simulink model "rls"  (R2022b)
settings: Solver=FixedStepAuto  StartTime=0.0  StopTime=910415*Ts  FixedStep=Ts  RelTol=1e-3
PreLoadFcn:
  | gen_workspace
undefined symbols (not defined in the file): Ts
settings Model: Creator=Z153167  LastModifiedBy=Z153167

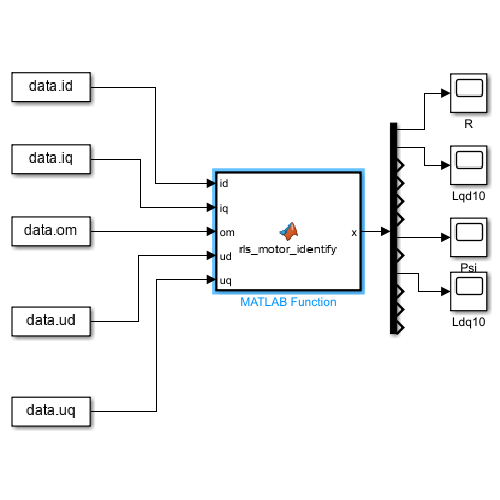
[thumbnail: Simulink's stored preview of the top-level diagram]
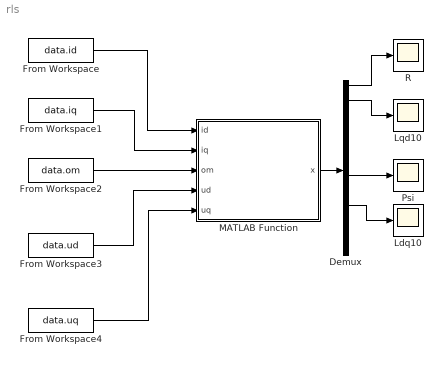
== system rls ==
  Demux : Demux  Outputs=12
  From Workspace : FromWorkspace  VariableName=data.id  SampleTime=Ts  OutputAfterFinalValue=Holding final value
  From Workspace1 : FromWorkspace  VariableName=data.iq  SampleTime=Ts  OutputAfterFinalValue=Holding final value
  From Workspace2 : FromWorkspace  VariableName=data.om  SampleTime=Ts  OutputAfterFinalValue=Holding final value
  From Workspace3 : FromWorkspace  VariableName=data.ud  SampleTime=Ts  OutputAfterFinalValue=Holding final value
  From Workspace4 : FromWorkspace  VariableName=data.uq  SampleTime=Ts  OutputAfterFinalValue=Holding final value
  Ldq10 : Scope
  Lqd10 : Scope
  MATLAB Function : MATLAB Function  TreatAsAtomicUnit=on
  Psi : Scope
  R : Scope
  wires:
  From Workspace2/1 -> MATLAB Function/3(om)
  From Workspace1/1 -> MATLAB Function/2(iq)
  From Workspace3/1 -> MATLAB Function/4(ud)
  From Workspace/1 -> MATLAB Function/1(id)
  From Workspace4/1 -> MATLAB Function/5(uq)
  MATLAB Function/1(x) -> Demux/1
  Demux/7 -> Psi/1
  Demux/1 -> R/1
  Demux/2 -> Lqd10/1
  Demux/9 -> Ldq10/1

== matlab function rls/MATLAB Function ==
  data: id input; x output; iq input; om input; ud input; uq input
function x = rls_motor_identify(id, iq, om, ud, uq)
% RLS_MOTOR_IDENTIFY  Rank-2 Recursive Least Squares parameter identification
%                     for a PMSM motor model, intended for use as a MATLAB
%                     Function block inside Simulink.
%
% USAGE (Simulink MATLAB Function block)
%   - Inputs  : id, iq, om, ud, uq  (all scalar, double)
%   - Output  : x  (12x1 double) — current parameter vector
%
% PARAMETER VECTOR  x  (12 elements, PARAMETER_NAMES order)
%   Index  Name      Axis
%   1      R         d
%   2      Lqd10     d
%   3      Lqd30     d
%   4      Cdq01     d
%   5      Cdq11     d
%   6      R         q   (= x(1) by constraint)
%   7      Psi       q
%   8      Cdq01     q   (= x(4) by constraint)
%   9      Ldq10     q
%   10     Ldq20     q
%   11     Ldq30     q
%   12     Cdq11     q   (= x(5) by constraint)
%
% EQUALITY CONSTRAINTS (enforced via null-space projection)
%   x(1)  == x(6)   (R shared between axes)
%   x(4)  == x(8)   (Cdq01 shared)
%   x(5)  == x(12)  (Cdq11 shared)
%
% ALGORITHM
%   At each time step the function performs one rank-2 RLS update using both
%   the d-axis (Ud) and q-axis (Uq) voltage equations simultaneously.
%   The Woodbury matrix identity is used so that only a cheap 2x2 matrix
%   inversion is required per step.
%   All arithmetic is carried out in the reduced (null-space) coordinate
%   system of dimension r = 9, then mapped back to the full 12-D space.
%
% PERSISTENT STATE
%   Minv  (9x9)  inverse of the reduced normal-equation matrix
%   rhs   (9x1)  reduced right-hand side  Ar' * b  accumulated so far
%   F     (12x9) null-space basis (fixed after first call)
%   x_    (12x1) current full-space parameter estimate

% -------------------------------------------------------------------------
% Persistent variables — survive across Simulink time steps.
% -------------------------------------------------------------------------
persistent Minv rhs F x_

% -------------------------------------------------------------------------
% Constants
% -------------------------------------------------------------------------
N_PARAMS = 12;

% Datasheet / prior-knowledge initial guesses.
start_values = [ ...
    3e-02;  50e-6;  0.;  0.;  0.; ...   % d-axis
    3e-02;  4e-03;  0.; 50e-6;  0.;  0.;  0.];  % q-axis

% Equality constraint pairs
% Each row is [i, j] meaning x(i) must equal x(j).
eq_pairs = [1, 6; 4, 8; 5, 12];  

% Number of synthetic initialisation samples.
N_INIT = 50;

% -------------------------------------------------------------------------
% One-time initialisation (first Simulink call or after a reset).
% -------------------------------------------------------------------------
if isempty(F)
    % --- Build null-space basis F (12 x 9) ---
    n_constraints = size(eq_pairs, 1);   % = 3
    C = zeros(n_constraints, N_PARAMS);
    for k = 1:n_constraints
        C(k, eq_pairs(k,1)) =  1;
        C(k, eq_pairs(k,2)) = -1;
    end
    % null() returns an orthonormal basis for the null space of C.
    F = null(C);   % (12 x 9)

    % --- Bootstrap cache from synthetic data ---
    % Replicate Python's initialise_cache: a linspace grid of 50 (id,iq,om)
    % samples.  The seed is fixed so the initial state is deterministic.
    rng(133);
    id_init  = linspace(-10, 10, N_INIT)' + randn(N_INIT, 1);
    iq_init  = linspace(-10, 10, N_INIT)' + randn(N_INIT, 1);
    om_init  = linspace(-100, 100, N_INIT)' + randn(N_INIT, 1);

    % Build the full (2*N_INIT x 12) design matrix A and target vector b.
    [b_init, A_init] = expand_basis_batch(id_init, iq_init, om_init, ...
                                          zeros(N_INIT,1), zeros(N_INIT,1));
    % Voltages consistent with start_values.
    b_init = A_init * start_values;

    % Project into the reduced space.
    Ar_init = A_init * F;           % (2*N_INIT x 9)
    Minv    = inv(Ar_init' * Ar_init);  % (9 x 9)
    rhs     = Ar_init' * b_init;        % (9 x 1)
    x_      = start_values;             % (12 x 1)
end

% -------------------------------------------------------------------------
% Build the two regressor rows for this time step.
% -------------------------------------------------------------------------
% d-axis row  (5 non-zero entries, columns 1-5):
%   [id,  -om*iq,  -om*iq^3,  -om*id*iq,  -0.5*om*iq*id^2,
%    0,    0,       0,          0,           0,              0, 0]
% q-axis row  (7 non-zero entries, columns 6-12):
%   [0,   0,        0,          0,           0,
%    iq,  om,  0.5*om*iq^2,  om*id,  om*id^2,  om*id^3,  0.5*om*id*iq^2]

a_d = [ id, ...
       -om*iq, ...
       -om*iq^3, ...
       -om*id*iq, ...
       -0.5*om*iq*id^2, ...
        0, 0, 0, 0, 0, 0, 0 ];       % (1 x 12)

a_q = [ 0, 0, 0, 0, 0, ...
        iq, ...
        om, ...
        0.5*om*iq^2, ...
        om*id, ...
        om*id^2, ...
        om*id^3, ...
        0.5*om*id*iq^2 ];             % (1 x 12)

A_new   = [a_d; a_q];        % (2 x 12)
b_new   = [ud; uq];          % (2 x 1)

% -------------------------------------------------------------------------
% Rank-2 RLS update in the reduced space (Woodbury identity).
% -------------------------------------------------------------------------
% Project the two new rows into the reduced space.
Ar_new   = F' * A_new';  % (9 x 2)     

Minv_U   = Minv * Ar_new; % (9 x 2) 

inner    = eye(2) + Ar_new' * Minv_U; % (2 x 2) 

% Explicit 2x2 inversion 
a_i = inner(1,1);  b_i = inner(1,2);
c_i = inner(2,1);  d_i = inner(2,2);
det_val = a_i*d_i - b_i*c_i;

if abs(det_val) < 1e-12
    % Near-singular: observation nearly collinear with existing data — skip.
    x = x_;
    return
end

inner_inv = [d_i, -b_i; -c_i, a_i] / det_val;   % (2 x 2)

% Woodbury update of the inverse.
Minv = Minv - Minv_U * inner_inv * Minv_U';      % (9 x 9)

% Update right-hand side and solve.
rhs  = rhs  + Ar_new * b_new;                    % (9 x 1)
xr   = Minv * rhs;                               % (9 x 1)

% Map back to the full 12-D parameter space.
x_   = F * xr;                                   % (12 x 1)
x    = x_;

end % function rls_motor_identify


% =========================================================================
%  LOCAL HELPER — batch basis expansion  (only used during initialisation)
% =========================================================================
function [b, A] = expand_basis_batch(id, iq, om, ud, uq)
% EXPAND_BASIS_BATCH  Assemble the (2N x 12) design matrix and (2N x 1)
%                     target vector for N samples.
%
% Rows are interleaved:  row 2k-1 → d-axis (Ud),  row 2k → q-axis (Uq).
% Column layout matches PARAMETER_NAMES (12 columns).

N = numel(id);
A = zeros(2*N, 12);

% d-axis columns (1-5), placed in odd rows (1,3,5,…):
A(1:2:end, 1) =  id;
A(1:2:end, 2) = -om .* iq;
A(1:2:end, 3) = -om .* iq.^3;
A(1:2:end, 4) = -om .* id .* iq;
A(1:2:end, 5) = -0.5 .* om .* iq .* id.^2;

% q-axis columns (6-12), placed in even rows (2,4,6,…):
A(2:2:end, 6)  =  iq;
A(2:2:end, 7)  =  om;
A(2:2:end, 8)  =  0.5 .* om .* iq.^2;
A(2:2:end, 9)  =  om .* id;
A(2:2:end, 10) =  om .* id.^2;
A(2:2:end, 11) =  om .* id.^3;
A(2:2:end, 12) =  0.5 .* om .* id .* iq.^2;

% Target voltages (interleaved Ud / Uq):
b = zeros(2*N, 1);
b(1:2:end) = ud;
b(2:2:end) = uq;
end
